simulink library "AP_RollController"  (R2024a)
settings: Solver=VariableStepAuto  StartTime=0.0  StopTime=10.0  RelTol=1e-3
undefined symbols (not defined in the file): RLL2SRV_TCONST, RLL_Freq, RLL_RATE_D, RLL_RATE_I, RLL_RATE_P
libraries: simulink_extras x4, ArdupilotFunctions x1
settings Model: Creator=igmso  LastModifiedBy=igmso

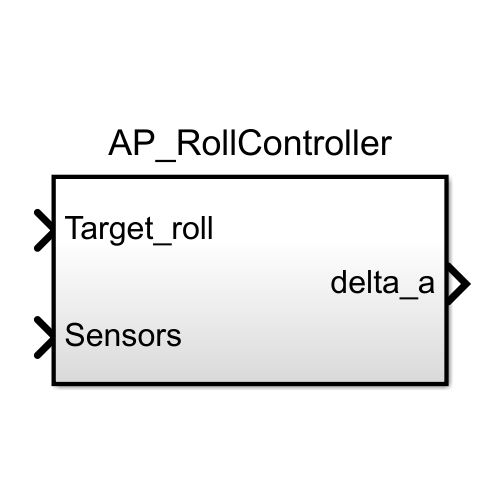
[thumbnail: Simulink's stored preview of the top-level diagram]
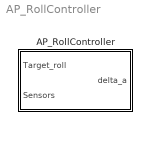
== system AP_RollController ==
  AP_RollController : Subsystem  TreatAsAtomicUnit=on  SystemSampleTime=1/RLL_Freq

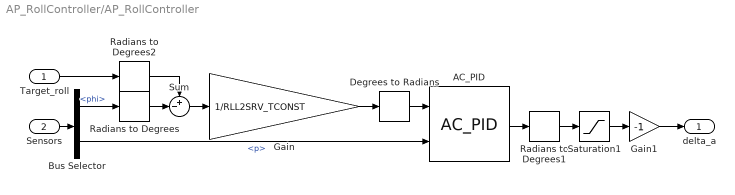
== system AP_RollController/AP_RollController ==
  Target_roll : Inport
  Sensors : Inport  Port=2
  AC_PID : ArdupilotFunctions/AC_PID  P=RLL_RATE_P  I=RLL_RATE_I  D=RLL_RATE_D  FF=RLL_RATE_FF  D_FF=RLL_RATE_D_FF  FLTD=RLL_RATE_FLTD  FLTE=RLL_RATE_FLTE  FLTT=RLL_RATE_FLTT  IMAX=RLL_RATE_IMAX  ControlFreq=RLL_Freq
  Bus Selector : BusSelector  OutputSignals=phi,p
  Degrees to Radians : simulink_extras/Transformations/Degrees to Radians
  Gain : Gain  Gain=1/RLL2SRV_TCONST
  Gain1 : Gain  Gain=-1
  Radians to Degrees : simulink_extras/Transformations/Radians to Degrees
  Radians to Degrees1 : simulink_extras/Transformations/Radians to Degrees
  Radians to Degrees2 : simulink_extras/Transformations/Radians to Degrees
  Saturation1 : Saturate  UpperLimit=45  LowerLimit=-45
  Sum : Sum  Inputs=+-|
  delta_a : Outport
  wires:
  Gain1/1 -> delta_a/1
  Radians to Degrees/1 -> Sum/2
  Degrees to Radians/1 -> AC_PID/1
  Sensors/1 -> Bus Selector/1
  Bus Selector/1 -> Radians to Degrees/1  "<phi>"
  Saturation1/1 -> Gain1/1
  Bus Selector/2 -> AC_PID/2  "<p>"
  AC_PID/1 -> Radians to Degrees1/1
  Sum/1 -> Gain/1
  Gain/1 -> Degrees to Radians/1
  Radians to Degrees2/1 -> Sum/1
  Radians to Degrees1/1 -> Saturation1/1
  Target_roll/1 -> Radians to Degrees2/1
